simulink model "Plant0"  (R2024a)
settings: Solver=VariableStepAuto  StartTime=0.0  StopTime=10.0  RelTol=1e-3
model workspace (MATLAB code in the model file):
  | WheelParams;
  | BodyParams;
  | SensorParams;
undefined symbols (not defined in the file): body_inertia, body_mass
settings Model: Creator=Marij  LastModifiedBy=Marij
settings OptimizationCC: UseDivisionForNetSlopeComputation=on
settings ModelReferenceCC: ModelReferenceMinAlgLoopOccurrences=on

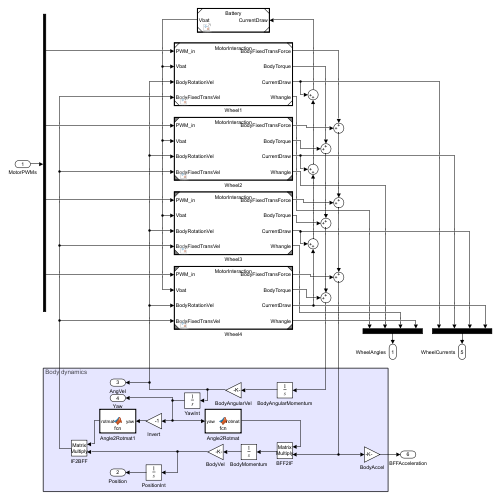
[thumbnail: Simulink's stored preview of the top-level diagram]
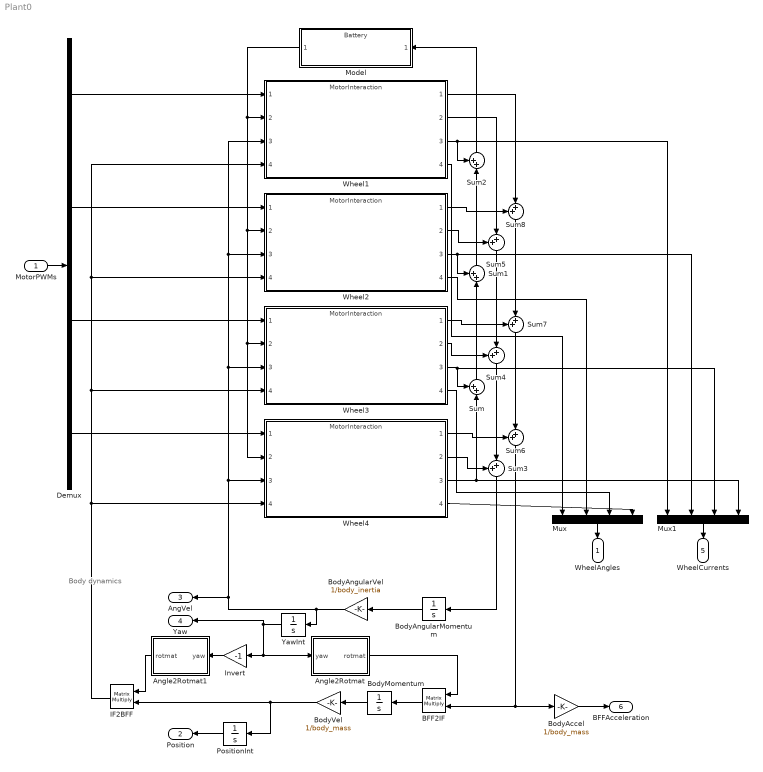
== system Plant0 ==
  note: Body dynamics
  MotorPWMs : Inport  PortDimensions=4
  Angle2Rotmat : MATLAB Function  TreatAsAtomicUnit=on
  Angle2Rotmat1 : MATLAB Function  TreatAsAtomicUnit=on
  BFF2IF : Product  Multiplication=Matrix(*)
  BodyAccel : Gain  Gain=1/body_mass
  BodyAngularMomentum : Integrator  ContinuousStateAttributes='AngularMomentum'
  BodyAngularVel : Gain  Gain=1/body_inertia
  BodyMomentum : Integrator  ContinuousStateAttributes={'XVelocity', 'YVelocity'}
  BodyVel : Gain  Gain=1/body_mass
  Demux : Demux
  IF2BFF : Product  Multiplication=Matrix(*)
  Invert : Gain  Gain=-1
  Model : ModelReference  ModelNameDialog=Battery.slx  SimulationMode=Normal  ModelReferenceVersion=1.2
  Mux : Mux
  Mux1 : Mux
  PositionInt : Integrator  ContinuousStateAttributes={'XPosition', 'YPosition'}
  Sum{,1..8} (9 alike) : Sum  Inputs=++|
  Wheel{1..4} (4 alike) : ModelReference  ModelNameDialog=MotorInteraction.slx  UsingDefaultArgumentValue=0  SimulationMode=Normal  ModelReferenceVersion=1.41
  YawInt : Integrator  ContinuousStateAttributes='Yaw'
  WheelAngles : Outport  Unit=rad  PortDimensions=4
  Position : Outport  Port=2  Unit=m  PortDimensions=2
  AngVel : Outport  Port=3  Unit=rad/s  PortDimensions=1
  Yaw : Outport  Port=4  Unit=rad  PortDimensions=1
  WheelCurrents : Outport  Port=5  Unit=A  PortDimensions=4
  BFFAcceleration : Outport  Port=6
  wires:
  MotorPWMs/1 -> Demux/1
  Demux/1 -> Wheel1/1
  Demux/4 -> Wheel4/1
  Demux/3 -> Wheel3/1
  Demux/2 -> Wheel2/1
  Sum/1 -> Sum1/2
  Wheel2/3 -> Mux1/2, Sum1/1
  Sum1/1 -> Sum2/2
  Wheel1/3 -> Mux1/1, Sum2/1
  Wheel3/3 -> Mux1/3, Sum/1
  Wheel4/3 -> Mux1/4, Sum/2
  Sum2/1 -> Model/1
  Model/1 -> Wheel1/2, Wheel4/2, Wheel3/2, Wheel2/2
  Wheel4/2 -> Sum3/1
  Wheel3/2 -> Sum4/1
  Sum4/1 -> Sum3/2
  Sum5/1 -> Sum4/2
  Wheel2/2 -> Sum5/1
  Wheel1/2 -> Sum5/2
  Sum3/1 -> BodyAngularMomentum/1
  BodyAngularMomentum/1 -> BodyAngularVel/1
  BodyAngularVel/1 -> YawInt/1, AngVel/1, Wheel4/3, Wheel2/3, Wheel1/3, Wheel3/3
  Wheel4/1 -> Sum6/1
  Wheel3/1 -> Sum7/1
  Sum7/1 -> Sum6/2
  Wheel2/1 -> Sum8/1
  Sum8/1 -> Sum7/2
  Wheel1/1 -> Sum8/2
  YawInt/1 -> Yaw/1, Angle2Rotmat/1(yaw), Invert/1
  Sum6/1 -> BodyAccel/1, BFF2IF/2
  Angle2Rotmat/1(rotmat) -> BFF2IF/1
  BFF2IF/1 -> BodyMomentum/1
  BodyMomentum/1 -> BodyVel/1
  Invert/1 -> Angle2Rotmat1/1(yaw)
  BodyVel/1 -> PositionInt/1, IF2BFF/2
  Angle2Rotmat1/1(rotmat) -> IF2BFF/1
  IF2BFF/1 -> Wheel4/4, Wheel3/4, Wheel2/4, Wheel1/4
  Wheel4/4 -> Mux/4
  Wheel3/4 -> Mux/3
  Wheel2/4 -> Mux/2
  Wheel1/4 -> Mux/1
  Mux/1 -> WheelAngles/1
  PositionInt/1 -> Position/1
  Mux1/1 -> WheelCurrents/1
  BodyAccel/1 -> BFFAcceleration/1

== matlab function Plant0/Angle2Rotmat ==
  data: yaw input; rotmat output
function rotmat = fcn(yaw)
rotmat = [cos(yaw), -sin(yaw); sin(yaw), cos(yaw)];

== matlab function Plant0/Angle2Rotmat1 ==
  data: yaw input; rotmat output
function rotmat = fcn(yaw)
rotmat = [cos(yaw), -sin(yaw); sin(yaw), cos(yaw)];
